simulink model "gimbal_test_2017_11_24"  (R2017a)
settings: Solver=ode14x  StartTime=0.0  StopTime=20  FixedStep=0.001  RelTol=1e-3  EnableMultiTasking=on
values from neighbouring files (symbols this model uses):
  m = MAG(:,3:5)    [acc_calibration_t1.m]
  s = tf('s')    [adaptive_control.m]    (also in constraints.m = 1e-19)
undefined symbols (not defined in the file or in its folder): sigbuilder_block, X, Y, Z
libraries: sm_lib x46, nesl_utility x35, simulink x7
(part 1 of 2)
settings Model: Creator=Chaohua Zhao  LastModifiedBy=Chaohua Zhao
settings DataIOCC: LimitDataPoints=on
settings OptimizationCC: LifeSpan=inf
settings DebuggingCC: AllowSymbolicDim=off  SFUnexpectedBacktrackingDiag=warning  SFNoUnconditionalDefaultTransitionDiag=warning  SFExecutionAtInitializationDiag=none
settings ModelReferenceCC: PropagateSignalLabelsOutOfModel=off
settings GRTTargetCC: TargetLangStandard=C89/C90 (ANSI)
settings ConfigComp: CovMetricSettings=dw  CovHtmlReporting=on  CovSaveCumulativeToWorkspaceVar=on  CovSaveSingleToWorkspaceVar=on  CovExternalEMLEnable=off
settings ConfigurationSet: Description=SimMechanics 2G

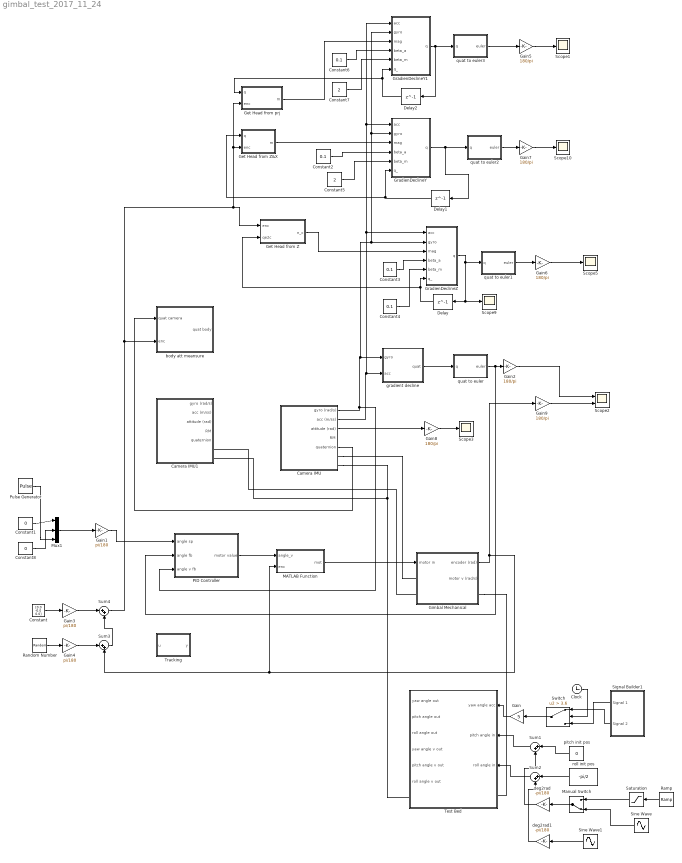
== system gimbal_test_2017_11_24 ==
  Camera IMU : Subsystem
  Camera IMU1 : Subsystem
  Clock : Clock
  Constant : Constant  Value=[0.0 -0.0 0.0]
  Constant1 : Constant  Value=0
  Constant{2..4,6} (4 alike) : Constant  Value=0.1
  Constant5 : Constant  Value=2
  Constant7 : Constant  Value=2
  Constant8 : Constant  Value=0
  Delay : Delay  DelayLength=1  InitialCondition=[1;0;0;0]
  Delay1 : Delay  DelayLength=1  InitialCondition=[1;0;0;0]
  Delay2 : Delay  DelayLength=1  InitialCondition=[1;0;0;0]
  Gain : Gain  Gain=5
  Gain1 : Gain  Gain=pi/180
  Gain{2,5..9} (6 alike) : Gain  Gain=180/pi
  Gain3 : Gain  Gain=pi/180
  Gain4 : Gain  Gain=pi/180
  Get Head from Z : MATLAB Function  TreatAsAtomicUnit=on
  Get Head from Z&X : MATLAB Function  TreatAsAtomicUnit=on
  "Get Head from prj " : MATLAB Function  TreatAsAtomicUnit=on
  Gimbal Mechanical : Subsystem
  GradienDeclineY : MATLAB Function  TreatAsAtomicUnit=on
  GradienDeclineY1 : MATLAB Function  TreatAsAtomicUnit=on
  GradienDeclineZ : MATLAB Function  TreatAsAtomicUnit=on
  MATLAB Function : MATLAB Function  TreatAsAtomicUnit=on
  Manual Switch : ManualSwitch  CurrentSetting=0
  Mux1 : Mux  Inputs=3
  PID Controller : Subsystem  TreatAsAtomicUnit=on
  Pulse Generator : DiscretePulseGenerator  PulseType=Time based  Amplitude=90  Period=3  PulseWidth=50
  Ramp : simulink/Sources/Ramp  slope=70  start=1  X0=0
  Random Number : RandomNumber  Variance=0.01  SampleTime=0.001
  Saturation : Saturate  UpperLimit=100  LowerLimit=-70
  Scope{1,3,5,9..10} (5 alike) : Scope
  Scope2 : Scope  NumInputPorts=2
  Signal Builder1 : Subsystem  Tag=STV Subsys  LoadFcn=sigbuilder_block('load');  StartFcn=sigbuilder_block('start');  StopFcn=sigbuilder_block('stop');  ClipboardFcn=sigbuilder_block('clipboard');  mask(Sigbuilder block){tuvar=[0:10]}
      mask help: Simulink:masks:SigbuilderBlock_MD
      mask init:
      | if ~strcmp(get_param(bdroot(gcbh),'SimulationStatus'),'stopped') tuvar = sigbuilder_block('maskInit'); end
      settings: CopyFcn=sigbuilder_block('copy');  DeleteFcn=sigbuilder_block('delete');  ModelCloseFcn=sigbuilder_block('modelClose');  PreSaveFcn=sigbuilder_block('preSave');  PauseFcn=sigbuilder_block('pause');  ContinueFcn=sigbuilder_block('continue');  NameChangeFcn=sigbuilder_block('namechange');  OpenFcn=sigbuilder_block('open',[6 74.25 1188 459 ]);  CloseFcn=sigbuilder_block('close');
      mask Display: plot(0, 0, 100, 100,[2, 2, 32, 32, 2], [68, 8, 8, 68, 68],[32, 2], [38, 38], [32, 19, 2],[53, 60, 44], [32, 17, 17, 2],[16, 16, 31, 31]);txt = getActiveGroup(gcbh);text(2, 100, txt,'verticalAlignment', 'top');
  Sine Wave : Sin  Amplitude=60  SampleTime=0
  Sine Wave1 : Sin  Amplitude=60  Frequency=1.7  SampleTime=0
  Sum{1..4} (4 alike) : Sum  Inputs=|++
  Switch : Switch  Criteria=u2 > Threshold  Threshold=3.6
  Test Bed : Subsystem
  Tracking : MATLAB Function  TreatAsAtomicUnit=on
  body att meansure : Subsystem
  deg2rad : Gain  Gain=-pi/180
  deg2rad1 : Gain  Gain=-pi/180
  gradient decline : Subsystem
  pitch init pos : Constant  Value=0
  quat to euler : MATLAB Function  TreatAsAtomicUnit=on
  quat to euler1 : MATLAB Function  TreatAsAtomicUnit=on
  quat to euler2 : MATLAB Function  TreatAsAtomicUnit=on
  quat to euler3 : MATLAB Function  TreatAsAtomicUnit=on
  roll init pos : Constant  Value=-pi/2
  wires:
  pitch init pos/1 -> Sum1/1
  roll init pos/1 -> Sum2/1
  Ramp/1 -> Saturation/1
  Saturation/1 -> Manual Switch/1
  Sine Wave/1 -> Manual Switch/2
  Manual Switch/1 -> deg2rad/1
  Clock/1 -> Switch/2
  Signal Builder1/2(Signal 2) -> Switch/1
  Signal Builder1/1(Signal 1) -> Switch/3
  Sum1/1 -> Test Bed/2(pitch angle in)
  Sum2/1 -> Test Bed/3(roll angle in)
  Sine Wave1/1 -> deg2rad1/1
  Gimbal Mechanical/1(encoder (rad)) -> Gain9/1, MATLAB Function/2(enc), Sum3/2
  Camera IMU/1(gyro (rad/s)) -> GradienDeclineY/2(gyro), GradienDeclineY1/2(gyro), GradienDeclineZ/2(gyro), gradient decline/1(gyro), PID Controller/3(angle v fb)
  Sum3/1 -> Sum4/2
  Constant/1 -> Gain3/1
  Gain3/1 -> Sum4/1
  Random Number/1 -> Gain4/1
  Gain4/1 -> Sum3/1
  Sum4/1 -> Get Head from Z/1(enc), "Get Head from prj "/2(enc), Get Head from Z&X/2(enc), body att meansure/2(enc)
  Camera IMU/2(acc (m/ss)) -> GradienDeclineY/1(acc), GradienDeclineY1/1(acc), GradienDeclineZ/1(acc), gradient decline/2(acc)
  gradient decline/1(quat) -> quat to euler/1(q)
  Camera IMU/5("quaternion ") -> body att meansure/1(quat camera)
  Gain1/1 -> PID Controller/1(angle sp)
  Gain2/1 -> Scope2/1
  GradienDeclineZ/1(q) -> quat to euler1/1(q), Delay/1, Scope9/1
  Delay/1 -> GradienDeclineZ/6(q_), Get Head from Z/2(qe2c)
  Constant3/1 -> GradienDeclineZ/4(beta_a)
  Switch/1 -> Gain/1
  Gain6/1 -> Scope5/1
  quat to euler1/1(euler) -> Gain6/1
  Get Head from Z/1(n_c) -> GradienDeclineZ/3(mag)
  Gain/1 -> Test Bed/1(yaw angle acc)
  Constant4/1 -> GradienDeclineZ/5(beta_m)
  Get Head from Z&X/1(m) -> GradienDeclineY/3(mag)
  Constant5/1 -> GradienDeclineY/5(beta_m)
  Constant2/1 -> GradienDeclineY/4(beta_a)
  Delay1/1 -> Get Head from Z&X/1(q), GradienDeclineY/6(q_)
  GradienDeclineY/1(q) -> quat to euler2/1(q), Delay1/1
  quat to euler2/1(euler) -> Gain7/1
  Gain7/1 -> Scope10/1
  quat to euler/1(euler) -> PID Controller/2(angle fb), Gain2/1
  "Get Head from prj "/1(m) -> GradienDeclineY1/3(mag)
  Constant6/1 -> GradienDeclineY1/4(beta_a)
  Constant7/1 -> GradienDeclineY1/5(beta_m)
  GradienDeclineY1/1(q) -> quat to euler3/1(q), Delay2/1
  Delay2/1 -> "Get Head from prj "/1(q), GradienDeclineY1/6(q_)
  Gain5/1 -> Scope1/1
  quat to euler3/1(euler) -> Gain5/1
  deg2rad/1 -> Sum1/2
  Gain8/1 -> Scope3/1
  Camera IMU/3(attitude (rad)) -> Gain8/1
  deg2rad1/1 -> Sum2/2
  Gain9/1 -> Scope2/2
  Constant1/1 -> Mux1/1
  Constant8/1 -> Mux1/2
  Pulse Generator/1 -> Mux1/3
  Mux1/1 -> Gain1/1
  PID Controller/1(motor value) -> MATLAB Function/1(angle_v)
  MATLAB Function/1(mot) -> Gimbal Mechanical/1(motor in)
  connections:
  Gimbal Mechanical/RConn1 -- Test Bed/LConn1
  Camera IMU/RConn1 -- Gimbal Mechanical/LConn1
  Camera IMU/RConn2 -- Camera IMU1/RConn2 -- Test Bed/RConn1
  Gimbal Mechanical/LConn2 -- Camera IMU1/RConn1

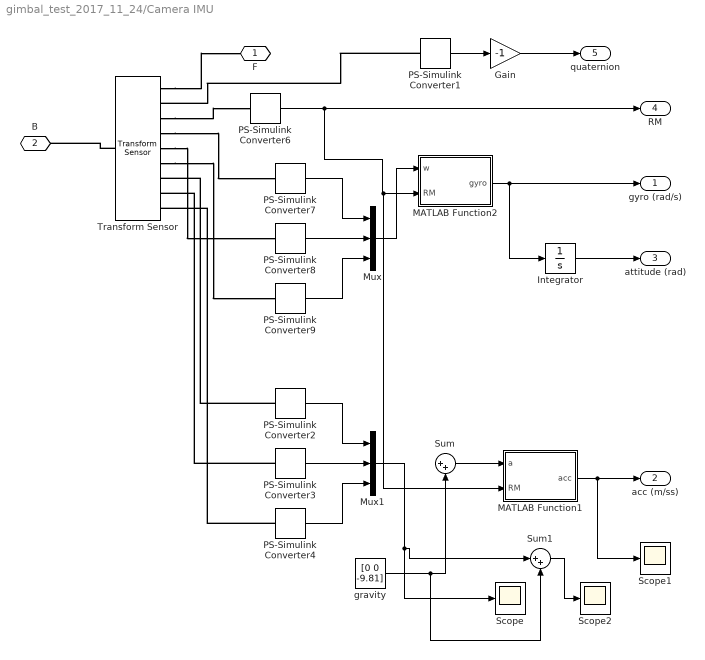
== system gimbal_test_2017_11_24/Camera IMU ==
  Gain : Gain  Gain=-1
  Integrator : Integrator
  MATLAB Function1 : MATLAB Function  TreatAsAtomicUnit=on
  MATLAB Function2 : MATLAB Function  TreatAsAtomicUnit=on
  Mux : Mux  Inputs=3
  Mux1 : Mux  Inputs=3
  PS-Simulink Converter{1..4,6..9} (8 alike) : nesl_utility/PS-Simulink Converter  PhysicalDomain=network_engine_domain  SubClassName=ps_output  LeftPortType=input  RightPortType=output  PseudoPeriodic=off  Frequencies=[]  Unit=1  AffineConversion=off
  Scope : Scope
  Scope1 : Scope
  Scope2 : Scope
  Sum : Sum  Inputs=|++
  Sum1 : Sum  Inputs=|++
  Transform Sensor : sm_lib/Frames and Transforms/Transform Sensor  MeasurementFrame=World  SenseAngle=off  SenseAxis=off  SenseAngle1=off  SenseAngle2=off  SenseAngle3=off  SenseQ=on  SenseR=on  SenseOmegaX=on  SenseOmegaY=on  SenseOmegaZ=on  SenseOmega1=off  SenseOmega2=off  SenseOmega3=off  SenseQDot=off  SenseRDot=off  SenseAlphaX=off  SenseAlphaY=off  SenseAlphaZ=off  SenseAlpha1=off  SenseAlpha2=off  SenseAlpha3=off  SenseQDDot=off  SenseRDDot=off  SenseX=off  SenseY=off  SenseZ=off  SenseRad=off  SenseAzim=off  SenseDist=off  SenseInc=off  SenseXDot=off  SenseYDot=off  SenseZDot=off  SenseRadDot=off  SenseAzimDot=off  SenseDistDot=off  SenseIncDot=off  SenseXDDot=on  SenseYDDot=on  SenseZDDot=on  SenseRadDDot=off  SenseAzimDDot=off  SenseDistDDot=off  SenseIncDDot=off
  "gravity " : Constant  Value=[0 0 -9.81]
  F : PMIOPort  Port=1  Side=Right
  B : PMIOPort  Port=2  Side=Right
  gyro (rad/s) : Outport
  acc (m/ss) : Outport  Port=2
  attitude (rad) : Outport  Port=3
  RM : Outport  Port=4
  "quaternion " : Outport  Port=5
  wires:
  PS-Simulink Converter6/1 -> RM/1, MATLAB Function1/2(RM), MATLAB Function2/2(RM)
  PS-Simulink Converter7/1 -> Mux/1
  PS-Simulink Converter9/1 -> Mux/3
  MATLAB Function2/1(gyro) -> gyro (rad/s)/1, Integrator/1
  PS-Simulink Converter8/1 -> Mux/2
  Integrator/1 -> attitude (rad)/1
  Mux/1 -> MATLAB Function2/1(w)
  PS-Simulink Converter1/1 -> Gain/1
  Gain/1 -> "quaternion "/1
  PS-Simulink Converter3/1 -> Mux1/2
  PS-Simulink Converter4/1 -> Mux1/3
  PS-Simulink Converter2/1 -> Mux1/1
  MATLAB Function1/1(acc) -> Scope1/1, acc (m/ss)/1
  "gravity "/1 -> Sum/2, Sum1/2
  Sum/1 -> MATLAB Function1/1(a)
  Sum1/1 -> Scope2/1
  Mux1/1 -> Sum1/1, Scope/1
  connections:
  Transform Sensor/LConn1 -- B/RConn1
  Transform Sensor/RConn1 -- F/RConn1
  Transform Sensor/RConn6 -- PS-Simulink Converter9/LConn1
  Transform Sensor/RConn5 -- PS-Simulink Converter8/LConn1
  Transform Sensor/RConn4 -- PS-Simulink Converter7/LConn1
  Transform Sensor/RConn3 -- PS-Simulink Converter6/LConn1
  PS-Simulink Converter1/LConn1 -- Transform Sensor/RConn2
  PS-Simulink Converter3/LConn1 -- Transform Sensor/RConn8
  PS-Simulink Converter4/LConn1 -- Transform Sensor/RConn9
  PS-Simulink Converter2/LConn1 -- Transform Sensor/RConn7

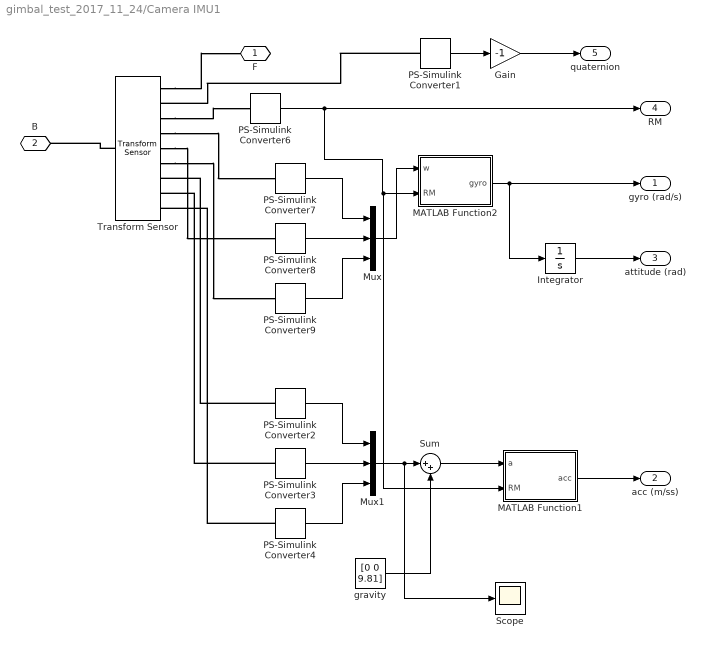
== system gimbal_test_2017_11_24/Camera IMU1 ==
  Gain : Gain  Gain=-1
  Integrator : Integrator
  MATLAB Function1 : MATLAB Function  TreatAsAtomicUnit=on
  MATLAB Function2 : MATLAB Function  TreatAsAtomicUnit=on
  Mux : Mux  Inputs=3
  Mux1 : Mux  Inputs=3
  PS-Simulink Converter{1..4,6..9} (8 alike) : nesl_utility/PS-Simulink Converter  PhysicalDomain=network_engine_domain  SubClassName=ps_output  LeftPortType=input  RightPortType=output  PseudoPeriodic=off  Frequencies=[]  Unit=1  AffineConversion=off
  Scope : Scope
  Sum : Sum  Inputs=|++
  Transform Sensor : sm_lib/Frames and Transforms/Transform Sensor  MeasurementFrame=World  SenseAngle=off  SenseAxis=off  SenseAngle1=off  SenseAngle2=off  SenseAngle3=off  SenseQ=on  SenseR=on  SenseOmegaX=on  SenseOmegaY=on  SenseOmegaZ=on  SenseOmega1=off  SenseOmega2=off  SenseOmega3=off  SenseQDot=off  SenseRDot=off  SenseAlphaX=off  SenseAlphaY=off  SenseAlphaZ=off  SenseAlpha1=off  SenseAlpha2=off  SenseAlpha3=off  SenseQDDot=off  SenseRDDot=off  SenseX=off  SenseY=off  SenseZ=off  SenseRad=off  SenseAzim=off  SenseDist=off  SenseInc=off  SenseXDot=off  SenseYDot=off  SenseZDot=off  SenseRadDot=off  SenseAzimDot=off  SenseDistDot=off  SenseIncDot=off  SenseXDDot=on  SenseYDDot=on  SenseZDDot=on  SenseRadDDot=off  SenseAzimDDot=off  SenseDistDDot=off  SenseIncDDot=off
  "gravity " : Constant  Value=[0 0 9.81]
  F : PMIOPort  Port=1  Side=Right
  B : PMIOPort  Port=2  Side=Right
  gyro (rad/s) : Outport
  acc (m/ss) : Outport  Port=2
  attitude (rad) : Outport  Port=3
  RM : Outport  Port=4
  "quaternion " : Outport  Port=5
  wires:
  Sum/1 -> MATLAB Function1/1(a)
  "gravity "/1 -> Sum/2
  Mux1/1 -> Sum/1, Scope/1
  MATLAB Function1/1(acc) -> acc (m/ss)/1
  PS-Simulink Converter2/1 -> Mux1/1
  PS-Simulink Converter4/1 -> Mux1/3
  PS-Simulink Converter3/1 -> Mux1/2
  Gain/1 -> "quaternion "/1
  PS-Simulink Converter1/1 -> Gain/1
  Mux/1 -> MATLAB Function2/1(w)
  Integrator/1 -> attitude (rad)/1
  PS-Simulink Converter8/1 -> Mux/2
  MATLAB Function2/1(gyro) -> Integrator/1, gyro (rad/s)/1
  PS-Simulink Converter9/1 -> Mux/3
  PS-Simulink Converter7/1 -> Mux/1
  PS-Simulink Converter6/1 -> MATLAB Function2/2(RM), MATLAB Function1/2(RM), RM/1
  connections:
  PS-Simulink Converter2/LConn1 -- Transform Sensor/RConn7
  PS-Simulink Converter4/LConn1 -- Transform Sensor/RConn9
  PS-Simulink Converter3/LConn1 -- Transform Sensor/RConn8
  PS-Simulink Converter1/LConn1 -- Transform Sensor/RConn2
  Transform Sensor/RConn3 -- PS-Simulink Converter6/LConn1
  Transform Sensor/RConn4 -- PS-Simulink Converter7/LConn1
  Transform Sensor/RConn5 -- PS-Simulink Converter8/LConn1
  Transform Sensor/RConn6 -- PS-Simulink Converter9/LConn1
  Transform Sensor/RConn1 -- F/RConn1
  Transform Sensor/LConn1 -- B/RConn1

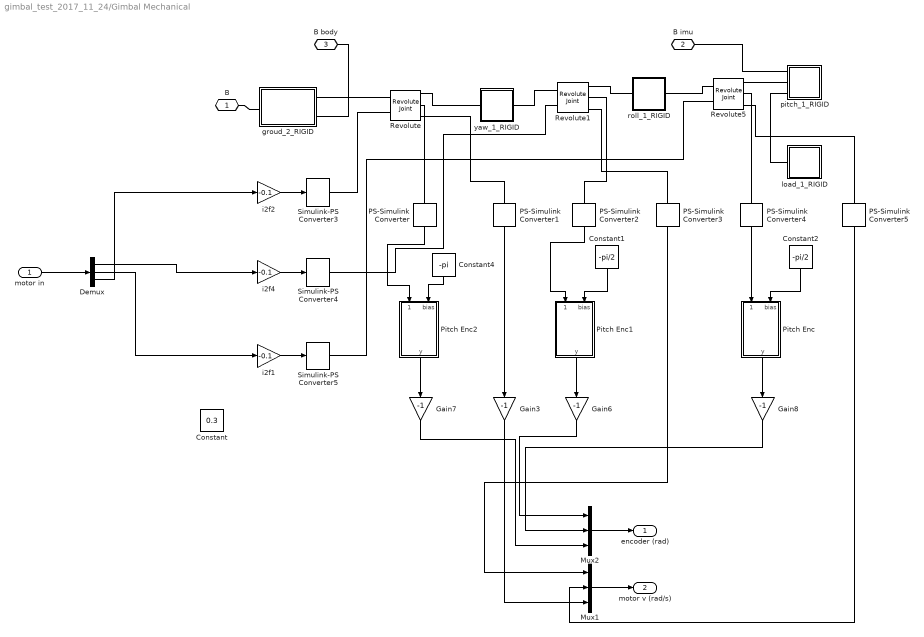
== system gimbal_test_2017_11_24/Gimbal Mechanical ==
  motor in : Inport
  Constant : Constant  Value=0.3
  Constant1 : Constant  Value=-pi/2
  Constant2 : Constant  Value=-pi/2
  Constant4 : Constant  Value=-pi
  Demux : Demux  Outputs=3
  Gain{3,6..8} (4 alike) : Gain  Gain=-1
  Mux1 : Mux  Inputs=3
  Mux2 : Mux  Inputs=3
  PS-Simulink Converter{,1..5} (6 alike) : nesl_utility/PS-Simulink Converter  PhysicalDomain=network_engine_domain  SubClassName=ps_output  LeftPortType=input  RightPortType=output  PseudoPeriodic=off  Frequencies=[]  Unit=1  AffineConversion=off
  Pitch Enc : MATLAB Function  TreatAsAtomicUnit=on
  Pitch Enc1 : MATLAB Function  TreatAsAtomicUnit=on
  Pitch Enc2 : MATLAB Function  TreatAsAtomicUnit=on
  Revolute : sm_lib/Joints/Revolute Joint  SenseConstraintForce=off  SenseConstraintForceX=off  SenseConstraintForceY=off  SenseConstraintForceZ=off  SenseConstraintTorque=off  SenseConstraintTorqueX=off  SenseConstraintTorqueY=off  SenseConstraintTorqueZ=off  SenseTotalForce=off  SenseTotalForceX=off  SenseTotalForceY=off  SenseTotalForceZ=off  SenseTotalTorque=off  SenseTotalTorqueX=off  SenseTotalTorqueY=off  SenseTotalTorqueZ=off  CompositeWrenchDir=FollowerOnBase  CompositeWrenchFrame=BaseFrame  EquilibriumPosition=0  EquilibriumPositionUnits=rad  SpringStiffness=0  SpringStiffnessUnits=m*N/rad  DampingCoefficient=0  DampingCoefficientUnits=m*s*N/rad  TorqueActuationMode=InputTorque  MotionActuationMode=ComputedMotion  SensePosition=on  SenseVelocity=on  SenseAcceleration=off  SenseTorqueForce=off  PositionTargetSpecify=on  PositionTargetPriority=Low  PositionTargetValue=180  PositionTargetValueUnits=deg  VelocityTargetSpecify=off  VelocityTargetPriority=High  VelocityTargetValue=0  VelocityTargetValueUnits=deg/s
  Revolute1 : sm_lib/Joints/Revolute Joint  SenseConstraintForce=off  SenseConstraintForceX=off  SenseConstraintForceY=off  SenseConstraintForceZ=off  SenseConstraintTorque=off  SenseConstraintTorqueX=off  SenseConstraintTorqueY=off  SenseConstraintTorqueZ=off  SenseTotalForce=off  SenseTotalForceX=off  SenseTotalForceY=off  SenseTotalForceZ=off  SenseTotalTorque=off  SenseTotalTorqueX=off  SenseTotalTorqueY=off  SenseTotalTorqueZ=off  CompositeWrenchDir=FollowerOnBase  CompositeWrenchFrame=BaseFrame  EquilibriumPosition=0  EquilibriumPositionUnits=rad  SpringStiffness=0  SpringStiffnessUnits=m*N/rad  DampingCoefficient=0  DampingCoefficientUnits=m*s*N/rad  TorqueActuationMode=InputTorque  MotionActuationMode=ComputedMotion  SensePosition=on  SenseVelocity=on  SenseAcceleration=off  SenseTorqueForce=off  PositionTargetSpecify=on  PositionTargetPriority=Low  PositionTargetValue=90  PositionTargetValueUnits=deg  VelocityTargetSpecify=off  VelocityTargetPriority=High  VelocityTargetValue=0  VelocityTargetValueUnits=deg/s
  Revolute5 : sm_lib/Joints/Revolute Joint  SenseConstraintForce=off  SenseConstraintForceX=off  SenseConstraintForceY=off  SenseConstraintForceZ=off  SenseConstraintTorque=off  SenseConstraintTorqueX=off  SenseConstraintTorqueY=off  SenseConstraintTorqueZ=off  SenseTotalForce=off  SenseTotalForceX=off  SenseTotalForceY=off  SenseTotalForceZ=off  SenseTotalTorque=off  SenseTotalTorqueX=off  SenseTotalTorqueY=off  SenseTotalTorqueZ=off  CompositeWrenchDir=FollowerOnBase  CompositeWrenchFrame=BaseFrame  EquilibriumPosition=0  EquilibriumPositionUnits=rad  SpringStiffness=0  SpringStiffnessUnits=m*N/rad  DampingCoefficient=0  DampingCoefficientUnits=m*s*N/rad  TorqueActuationMode=InputTorque  MotionActuationMode=ComputedMotion  SensePosition=on  SenseVelocity=on  SenseAcceleration=off  SenseTorqueForce=off  PositionTargetSpecify=on  PositionTargetPriority=Low  PositionTargetValue=90  PositionTargetValueUnits=deg  VelocityTargetSpecify=off  VelocityTargetPriority=High  VelocityTargetValue=0  VelocityTargetValueUnits=deg/s
  Simulink-PS Converter3 : nesl_utility/Simulink-PS Converter  PhysicalDomain=network_engine_domain  SubClassName=ps_input  LeftPortType=input  RightPortType=output  PseudoPeriodic=off  Frequencies=[]  NoiseDistribution=none  NoiseParameters=[]  Unit=1  AffineConversion=off  FilteringAndDerivatives=zero  SimscapeFilterOrder=1  InputFilterTimeConstant=0.001  UdotUserProvided=1
  Simulink-PS Converter4 : nesl_utility/Simulink-PS Converter  PhysicalDomain=network_engine_domain  SubClassName=ps_input  LeftPortType=input  RightPortType=output  PseudoPeriodic=off  Frequencies=[]  NoiseDistribution=none  NoiseParameters=[]  Unit=1  AffineConversion=off  FilteringAndDerivatives=zero  SimscapeFilterOrder=1  InputFilterTimeConstant=0.001  UdotUserProvided=1
  Simulink-PS Converter5 : nesl_utility/Simulink-PS Converter  PhysicalDomain=network_engine_domain  SubClassName=ps_input  LeftPortType=input  RightPortType=output  PseudoPeriodic=off  Frequencies=[]  NoiseDistribution=none  NoiseParameters=[]  Unit=1  AffineConversion=off  FilteringAndDerivatives=zero  SimscapeFilterOrder=1  InputFilterTimeConstant=0.001  UdotUserProvided=1
  groud_2_RIGID : Subsystem
  i2f1 : Gain  Gain=-0.1
  i2f2 : Gain  Gain=-0.1
  i2f4 : Gain  Gain=-0.1
  load_1_RIGID : Subsystem
  pitch_1_RIGID : Subsystem
  roll_1_RIGID : Subsystem
  yaw_1_RIGID : Subsystem
  B : PMIOPort  Port=1  Side=Right
  B imu : PMIOPort  Port=2  Side=Left
  B body : PMIOPort  Port=3  Side=Left
  encoder (rad) : Outport
  motor v (rad/s) : Outport  Port=2
  wires:
  PS-Simulink Converter5/1 -> Mux1/2
  PS-Simulink Converter2/1 -> Pitch Enc1/1(angle)
  Constant1/1 -> Pitch Enc1/2(bias)
  Constant4/1 -> Pitch Enc2/2(bias)
  PS-Simulink Converter1/1 -> Gain3/1
  Constant2/1 -> Pitch Enc/2(bias)
  PS-Simulink Converter/1 -> Pitch Enc2/1(angle)
  PS-Simulink Converter4/1 -> Pitch Enc/1(angle)
  Pitch Enc1/1(y) -> Gain6/1
  Pitch Enc/1(y) -> Gain8/1
  PS-Simulink Converter3/1 -> Mux1/1
  Pitch Enc2/1(y) -> Gain7/1
  Gain7/1 -> Mux2/3
  Gain8/1 -> Mux2/2
  i2f4/1 -> Simulink-PS Converter4/1
  i2f1/1 -> Simulink-PS Converter5/1
  i2f2/1 -> Simulink-PS Converter3/1
  Gain6/1 -> Mux2/1
  ? -> ?
  Mux2/1 -> encoder (rad)/1
  Mux1/1 -> motor v (rad/s)/1
  Gain3/1 -> Mux1/3
  motor in/1 -> Demux/1
  Demux/1 -> i2f4/1
  Demux/2 -> i2f1/1
  Demux/3 -> i2f2/1
  connections:
  Revolute5/RConn1 -- pitch_1_RIGID/LConn2
  Revolute1/LConn1 -- yaw_1_RIGID/RConn1
  Revolute1/RConn1 -- roll_1_RIGID/LConn1
  Revolute/LConn1 -- groud_2_RIGID/RConn1
  groud_2_RIGID/LConn1 -- B/RConn1
  Revolute/RConn1 -- yaw_1_RIGID/LConn1
  load_1_RIGID/LConn1 -- pitch_1_RIGID/LConn3
  Revolute5/LConn1 -- roll_1_RIGID/RConn1
  Simulink-PS Converter5/RConn1 -- Revolute5/LConn2
  PS-Simulink Converter4/LConn1 -- Revolute5/RConn2
  PS-Simulink Converter5/LConn1 -- Revolute5/RConn3
  PS-Simulink Converter/LConn1 -- Revolute/RConn2
  PS-Simulink Converter3/LConn1 -- Revolute1/RConn3
  PS-Simulink Converter2/LConn1 -- Revolute1/RConn2
  PS-Simulink Converter1/LConn1 -- Revolute/RConn3
  Simulink-PS Converter3/RConn1 -- Revolute/LConn2
  Simulink-PS Converter4/RConn1 -- Revolute1/LConn2
  B imu/RConn1 -- pitch_1_RIGID/LConn1
  groud_2_RIGID/RConn2 -- B body/RConn1

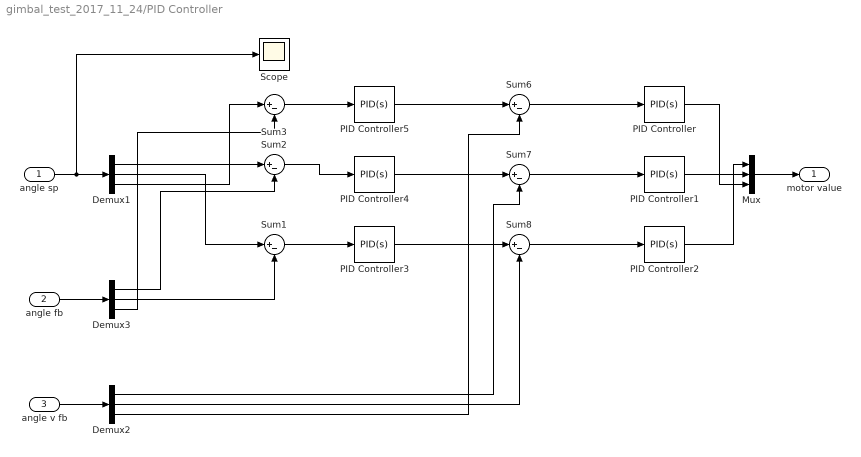
== system gimbal_test_2017_11_24/PID Controller ==
  angle sp : Inport
  angle fb : Inport  Port=2
  angle v fb : Inport  Port=3
  Demux1 : Demux  Outputs=3
  Demux2 : Demux  Outputs=3
  Demux3 : Demux  Outputs=3
  Mux : Mux  Inputs=3
  PID Controller : simulink/Continuous/PID Controller  Controller=PID  TimeDomain=Continuous-time  SampleTime=-1  IntegratorMethod=Forward Euler  FilterMethod=Forward Euler  Form=Parallel  UseFilter=on  ControllerParametersSource=internal  P=50  I=2  D=0.5  N=1  InitialConditionSource=internal  InitialConditionForIntegrator=0  InitialConditionForFilter=0  ExternalReset=none  LimitOutput=on  UpperSaturationLimit=10  LowerSaturationLimit=-10  LinearizeAsGain=on  AntiWindupMode=none  Kb=1  TrackingMode=off  Kt=1  PParamMin=[]  PParamMax=[]  IParamMin=[]  IParamMax=[]  DParamMin=[]  DParamMax=[]  NParamMin=[]  NParamMax=[]  KbParamMin=[]  KbParamMax=[]  KtParamMin=[]  KtParamMax=[]  POutMin=[]  POutMax=[]  IOutMin=[]  IOutMax=[]  DOutMin=[]  DOutMax=[]  NOutMin=[]  NOutMax=[]  KbOutMin=[]  KbOutMax=[]  KtOutMin=[]  KtOutMax=[]  IntegratorOutMin=[]  IntegratorOutMax=[]  FilterOutMin=[]  FilterOutMax=[]  SumOutMin=[]  SumOutMax=[]  SumI1OutMin=[]  SumI1OutMax=[]  SumI2OutMin=[]  SumI2OutMax=[]  SumI3OutMin=[]  SumI3OutMax=[]  SumDOutMin=[]  SumDOutMax=[]  SaturationOutMin=[]  SaturationOutMax=[]  IntegratorContinuousStateAttributes=''  IntegratorStateMustResolveToSignalObject=off  IntegratorRTWStateStorageClass=Auto  FilterContinuousStateAttributes=''  FilterStateMustResolveToSignalObject=off  FilterRTWStateStorageClass=Auto  DifferentiatorICPrevScaledInput=0  DifferentiatorOutMin=[]  DifferentiatorOutMax=[]  InitialConditionSetting=State (most efficient)
  PID Controller1 : simulink/Continuous/PID Controller  Controller=PID  TimeDomain=Continuous-time  SampleTime=-1  IntegratorMethod=Forward Euler  FilterMethod=Forward Euler  Form=Parallel  UseFilter=on  ControllerParametersSource=internal  P=50  I=2  D=0.5  N=20  InitialConditionSource=internal  InitialConditionForIntegrator=0  InitialConditionForFilter=0  ExternalReset=none  LimitOutput=on  UpperSaturationLimit=10  LowerSaturationLimit=-10  LinearizeAsGain=on  AntiWindupMode=none  Kb=1  TrackingMode=off  Kt=1  PParamMin=[]  PParamMax=[]  IParamMin=[]  IParamMax=[]  DParamMin=[]  DParamMax=[]  NParamMin=[]  NParamMax=[]  KbParamMin=[]  KbParamMax=[]  KtParamMin=[]  KtParamMax=[]  POutMin=[]  POutMax=[]  IOutMin=[]  IOutMax=[]  DOutMin=[]  DOutMax=[]  NOutMin=[]  NOutMax=[]  KbOutMin=[]  KbOutMax=[]  KtOutMin=[]  KtOutMax=[]  IntegratorOutMin=[]  IntegratorOutMax=[]  FilterOutMin=[]  FilterOutMax=[]  SumOutMin=[]  SumOutMax=[]  SumI1OutMin=[]  SumI1OutMax=[]  SumI2OutMin=[]  SumI2OutMax=[]  SumI3OutMin=[]  SumI3OutMax=[]  SumDOutMin=[]  SumDOutMax=[]  SaturationOutMin=[]  SaturationOutMax=[]  IntegratorContinuousStateAttributes=''  IntegratorStateMustResolveToSignalObject=off  IntegratorRTWStateStorageClass=Auto  FilterContinuousStateAttributes=''  FilterStateMustResolveToSignalObject=off  FilterRTWStateStorageClass=Auto  DifferentiatorICPrevScaledInput=0  DifferentiatorOutMin=[]  DifferentiatorOutMax=[]  InitialConditionSetting=State (most efficient)
  PID Controller2 : simulink/Continuous/PID Controller  Controller=PID  TimeDomain=Continuous-time  SampleTime=-1  IntegratorMethod=Forward Euler  FilterMethod=Forward Euler  Form=Parallel  UseFilter=on  ControllerParametersSource=internal  P=50  I=0.4  D=0.5  N=20  InitialConditionSource=internal  InitialConditionForIntegrator=0  InitialConditionForFilter=0  ExternalReset=none  LimitOutput=on  UpperSaturationLimit=10  LowerSaturationLimit=-10  LinearizeAsGain=on  AntiWindupMode=none  Kb=1  TrackingMode=off  Kt=1  PParamMin=[]  PParamMax=[]  IParamMin=[]  IParamMax=[]  DParamMin=[]  DParamMax=[]  NParamMin=[]  NParamMax=[]  KbParamMin=[]  KbParamMax=[]  KtParamMin=[]  KtParamMax=[]  POutMin=[]  POutMax=[]  IOutMin=[]  IOutMax=[]  DOutMin=[]  DOutMax=[]  NOutMin=[]  NOutMax=[]  KbOutMin=[]  KbOutMax=[]  KtOutMin=[]  KtOutMax=[]  IntegratorOutMin=[]  IntegratorOutMax=[]  FilterOutMin=[]  FilterOutMax=[]  SumOutMin=[]  SumOutMax=[]  SumI1OutMin=[]  SumI1OutMax=[]  SumI2OutMin=[]  SumI2OutMax=[]  SumI3OutMin=[]  SumI3OutMax=[]  SumDOutMin=[]  SumDOutMax=[]  SaturationOutMin=[]  SaturationOutMax=[]  IntegratorContinuousStateAttributes=''  IntegratorStateMustResolveToSignalObject=off  IntegratorRTWStateStorageClass=Auto  FilterContinuousStateAttributes=''  FilterStateMustResolveToSignalObject=off  FilterRTWStateStorageClass=Auto  DifferentiatorICPrevScaledInput=0  DifferentiatorOutMin=[]  DifferentiatorOutMax=[]  InitialConditionSetting=State (most efficient)
  PID Controller3 : simulink/Continuous/PID Controller  Controller=PID  TimeDomain=Continuous-time  SampleTime=-1  IntegratorMethod=Forward Euler  FilterMethod=Forward Euler  Form=Parallel  UseFilter=on  ControllerParametersSource=internal  P=10  I=0  D=0  N=20  InitialConditionSource=internal  InitialConditionForIntegrator=0  InitialConditionForFilter=0  ExternalReset=none  LimitOutput=on  UpperSaturationLimit=6  LowerSaturationLimit=-6  LinearizeAsGain=on  AntiWindupMode=none  Kb=1  TrackingMode=off  Kt=1  PParamMin=[]  PParamMax=[]  IParamMin=[]  IParamMax=[]  DParamMin=[]  DParamMax=[]  NParamMin=[]  NParamMax=[]  KbParamMin=[]  KbParamMax=[]  KtParamMin=[]  KtParamMax=[]  POutMin=[]  POutMax=[]  IOutMin=[]  IOutMax=[]  DOutMin=[]  DOutMax=[]  NOutMin=[]  NOutMax=[]  KbOutMin=[]  KbOutMax=[]  KtOutMin=[]  KtOutMax=[]  IntegratorOutMin=[]  IntegratorOutMax=[]  FilterOutMin=[]  FilterOutMax=[]  SumOutMin=[]  SumOutMax=[]  SumI1OutMin=[]  SumI1OutMax=[]  SumI2OutMin=[]  SumI2OutMax=[]  SumI3OutMin=[]  SumI3OutMax=[]  SumDOutMin=[]  SumDOutMax=[]  SaturationOutMin=[]  SaturationOutMax=[]  IntegratorContinuousStateAttributes=''  IntegratorStateMustResolveToSignalObject=off  IntegratorRTWStateStorageClass=Auto  FilterContinuousStateAttributes=''  FilterStateMustResolveToSignalObject=off  FilterRTWStateStorageClass=Auto  DifferentiatorICPrevScaledInput=0  DifferentiatorOutMin=[]  DifferentiatorOutMax=[]  InitialConditionSetting=State (most efficient)
  PID Controller4 : simulink/Continuous/PID Controller  Controller=PID  TimeDomain=Continuous-time  SampleTime=-1  IntegratorMethod=Forward Euler  FilterMethod=Forward Euler  Form=Parallel  UseFilter=on  ControllerParametersSource=internal  P=10  I=0  D=0  N=20  InitialConditionSource=internal  InitialConditionForIntegrator=0  InitialConditionForFilter=0  ExternalReset=none  LimitOutput=on  UpperSaturationLimit=6  LowerSaturationLimit=-6  LinearizeAsGain=on  AntiWindupMode=none  Kb=1  TrackingMode=off  Kt=1  PParamMin=[]  PParamMax=[]  IParamMin=[]  IParamMax=[]  DParamMin=[]  DParamMax=[]  NParamMin=[]  NParamMax=[]  KbParamMin=[]  KbParamMax=[]  KtParamMin=[]  KtParamMax=[]  POutMin=[]  POutMax=[]  IOutMin=[]  IOutMax=[]  DOutMin=[]  DOutMax=[]  NOutMin=[]  NOutMax=[]  KbOutMin=[]  KbOutMax=[]  KtOutMin=[]  KtOutMax=[]  IntegratorOutMin=[]  IntegratorOutMax=[]  FilterOutMin=[]  FilterOutMax=[]  SumOutMin=[]  SumOutMax=[]  SumI1OutMin=[]  SumI1OutMax=[]  SumI2OutMin=[]  SumI2OutMax=[]  SumI3OutMin=[]  SumI3OutMax=[]  SumDOutMin=[]  SumDOutMax=[]  SaturationOutMin=[]  SaturationOutMax=[]  IntegratorContinuousStateAttributes=''  IntegratorStateMustResolveToSignalObject=off  IntegratorRTWStateStorageClass=Auto  FilterContinuousStateAttributes=''  FilterStateMustResolveToSignalObject=off  FilterRTWStateStorageClass=Auto  DifferentiatorICPrevScaledInput=0  DifferentiatorOutMin=[]  DifferentiatorOutMax=[]  InitialConditionSetting=State (most efficient)
  PID Controller5 : simulink/Continuous/PID Controller  Controller=PID  TimeDomain=Continuous-time  SampleTime=-1  IntegratorMethod=Forward Euler  FilterMethod=Forward Euler  Form=Parallel  UseFilter=on  ControllerParametersSource=internal  P=10  I=0  D=0  N=1  InitialConditionSource=internal  InitialConditionForIntegrator=0  InitialConditionForFilter=0  ExternalReset=none  LimitOutput=on  UpperSaturationLimit=6  LowerSaturationLimit=-6  LinearizeAsGain=on  AntiWindupMode=none  Kb=1  TrackingMode=off  Kt=1  PParamMin=[]  PParamMax=[]  IParamMin=[]  IParamMax=[]  DParamMin=[]  DParamMax=[]  NParamMin=[]  NParamMax=[]  KbParamMin=[]  KbParamMax=[]  KtParamMin=[]  KtParamMax=[]  POutMin=[]  POutMax=[]  IOutMin=[]  IOutMax=[]  DOutMin=[]  DOutMax=[]  NOutMin=[]  NOutMax=[]  KbOutMin=[]  KbOutMax=[]  KtOutMin=[]  KtOutMax=[]  IntegratorOutMin=[]  IntegratorOutMax=[]  FilterOutMin=[]  FilterOutMax=[]  SumOutMin=[]  SumOutMax=[]  SumI1OutMin=[]  SumI1OutMax=[]  SumI2OutMin=[]  SumI2OutMax=[]  SumI3OutMin=[]  SumI3OutMax=[]  SumDOutMin=[]  SumDOutMax=[]  SaturationOutMin=[]  SaturationOutMax=[]  IntegratorContinuousStateAttributes=''  IntegratorStateMustResolveToSignalObject=off  IntegratorRTWStateStorageClass=Auto  FilterContinuousStateAttributes=''  FilterStateMustResolveToSignalObject=off  FilterRTWStateStorageClass=Auto  DifferentiatorICPrevScaledInput=0  DifferentiatorOutMin=[]  DifferentiatorOutMax=[]  InitialConditionSetting=State (most efficient)
  Scope : Scope
  Sum{1..3,6..8} (6 alike) : Sum  Inputs=|+-
  motor value : Outport
  wires:
  Demux2/2 -> Sum8/2
  Sum7/1 -> PID Controller1/1
  Demux2/3 -> Sum6/2
  Sum8/1 -> PID Controller2/1
  Demux2/1 -> Sum7/2
  Sum6/1 -> PID Controller/1
  PID Controller2/1 -> Mux/2
  PID Controller/1 -> Mux/3
  angle v fb/1 -> Demux2/1
  Mux/1 -> motor value/1
  PID Controller1/1 -> Mux/1
  angle sp/1 -> Scope/1, Demux1/1
  PID Controller5/1 -> Sum6/1
  PID Controller4/1 -> Sum7/1
  PID Controller3/1 -> Sum8/1
  Demux1/3 -> Sum3/1
  Sum3/1 -> PID Controller5/1
  Demux1/1 -> Sum2/1
  Sum2/1 -> PID Controller4/1
  Demux1/2 -> Sum1/1
  Sum1/1 -> PID Controller3/1
  Demux3/1 -> Sum2/2
  Demux3/2 -> Sum1/2
  Demux3/3 -> Sum3/2
  angle fb/1 -> Demux3/1

== system gimbal_test_2017_11_24/Signal Builder1 ==
  Demux : Demux  Tag=STV Demux  Outputs=2
  FromWs : FromWorkspace  Tag=STV FromWs  VariableName=tuvar  SampleTime=0
      SigBuilderData=|
      | common.afterFinalStr = 'Extrapolate'
      | common.sampleTime = 0
      | dataSet.timeRange = [0 10]
      | dataSet.name = 'Group 1'
      | sbobj.Groups.Name = 'Group 1'
      | sbobj.Groups.Signals(1).Name = 'Signal 1'
      | sbobj.Groups.Signals(1).XData = [0 2.9 3.1 3.2 3.4 10]
      | sbobj.Groups.Signals(1).YData = [0 0 1 1 -0.005 0]
      | sbobj.Groups.Signals(2).Name = 'Signal 2'
      | sbobj.Groups.Signals(2).XData = [0 3.9 4.1 4.2 4.4 10]
      | sbobj.Groups.Signals(2).YData = [0 0 -1 -1 0 0]
  Signal 1 : Outport  Tag=STV Outport
  Signal 2 : Outport  Tag=STV Outport  Port=2
  wires:
  Demux/1 -> Signal 1/1
  FromWs/1 -> Demux/1
  Demux/2 -> Signal 2/1

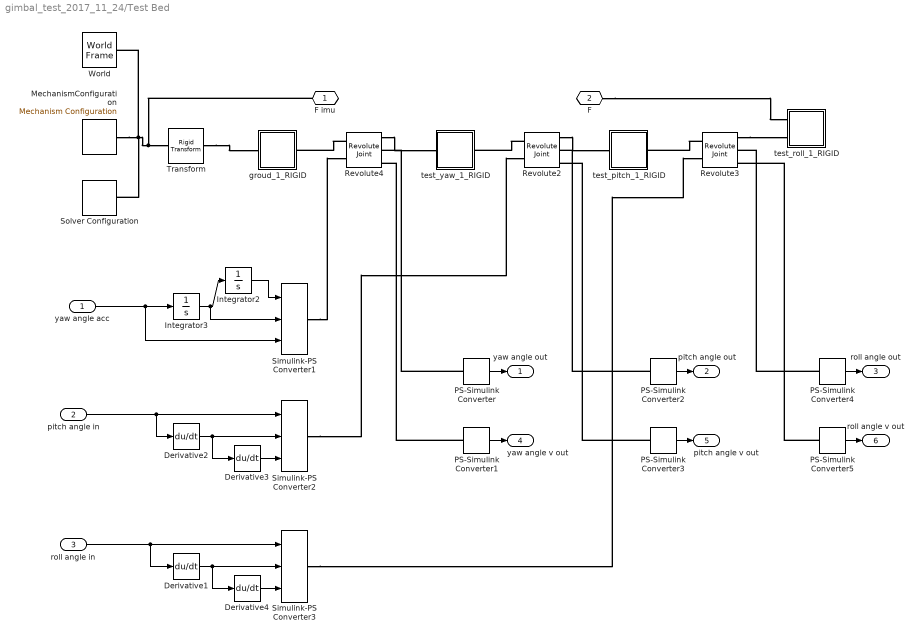
== system gimbal_test_2017_11_24/Test Bed ==
  yaw angle acc : Inport
  pitch angle in : Inport  Port=2
  roll angle in : Inport  Port=3
  Derivative{1..4} (4 alike) : Derivative
  Integrator2 : Integrator
  Integrator3 : Integrator
  MechanismConfiguration : sm_lib/Utilities/Mechanism Configuration  UniformGravity=Constant  GravityVector=[0 0 -9.81]  GravityUnits=m/s^2  LinearizationDelta=0.001
  PS-Simulink Converter{,1..5} (6 alike) : nesl_utility/PS-Simulink Converter  PhysicalDomain=network_engine_domain  SubClassName=ps_output  LeftPortType=input  RightPortType=output  PseudoPeriodic=off  Frequencies=[]  Unit=1  AffineConversion=off
  Revolute2 : sm_lib/Joints/Revolute Joint  SenseConstraintForce=off  SenseConstraintForceX=off  SenseConstraintForceY=off  SenseConstraintForceZ=off  SenseConstraintTorque=off  SenseConstraintTorqueX=off  SenseConstraintTorqueY=off  SenseConstraintTorqueZ=off  SenseTotalForce=off  SenseTotalForceX=off  SenseTotalForceY=off  SenseTotalForceZ=off  SenseTotalTorque=off  SenseTotalTorqueX=off  SenseTotalTorqueY=off  SenseTotalTorqueZ=off  CompositeWrenchDir=FollowerOnBase  CompositeWrenchFrame=BaseFrame  EquilibriumPosition=0  EquilibriumPositionUnits=rad  SpringStiffness=0  SpringStiffnessUnits=m*N/rad  DampingCoefficient=0  DampingCoefficientUnits=m*s*N/rad  TorqueActuationMode=ComputedTorque  MotionActuationMode=InputMotion  SensePosition=on  SenseVelocity=on  SenseAcceleration=off  SenseTorqueForce=off  PositionTargetSpecify=off  PositionTargetPriority=High  PositionTargetValue=0  PositionTargetValueUnits=deg  VelocityTargetSpecify=off  VelocityTargetPriority=High  VelocityTargetValue=0  VelocityTargetValueUnits=deg/s
  Revolute3 : sm_lib/Joints/Revolute Joint  SenseConstraintForce=off  SenseConstraintForceX=off  SenseConstraintForceY=off  SenseConstraintForceZ=off  SenseConstraintTorque=off  SenseConstraintTorqueX=off  SenseConstraintTorqueY=off  SenseConstraintTorqueZ=off  SenseTotalForce=off  SenseTotalForceX=off  SenseTotalForceY=off  SenseTotalForceZ=off  SenseTotalTorque=off  SenseTotalTorqueX=off  SenseTotalTorqueY=off  SenseTotalTorqueZ=off  CompositeWrenchDir=FollowerOnBase  CompositeWrenchFrame=BaseFrame  EquilibriumPosition=0  EquilibriumPositionUnits=rad  SpringStiffness=0  SpringStiffnessUnits=m*N/rad  DampingCoefficient=0  DampingCoefficientUnits=m*s*N/rad  TorqueActuationMode=ComputedTorque  MotionActuationMode=InputMotion  SensePosition=on  SenseVelocity=on  SenseAcceleration=off  SenseTorqueForce=off  PositionTargetSpecify=on  PositionTargetPriority=Low  PositionTargetValue=70.269058625743583  PositionTargetValueUnits=deg  VelocityTargetSpecify=off  VelocityTargetPriority=High  VelocityTargetValue=0  VelocityTargetValueUnits=deg/s
  Revolute4 : sm_lib/Joints/Revolute Joint  SenseConstraintForce=off  SenseConstraintForceX=off  SenseConstraintForceY=off  SenseConstraintForceZ=off  SenseConstraintTorque=off  SenseConstraintTorqueX=off  SenseConstraintTorqueY=off  SenseConstraintTorqueZ=off  SenseTotalForce=off  SenseTotalForceX=off  SenseTotalForceY=off  SenseTotalForceZ=off  SenseTotalTorque=off  SenseTotalTorqueX=off  SenseTotalTorqueY=off  SenseTotalTorqueZ=off  CompositeWrenchDir=FollowerOnBase  CompositeWrenchFrame=BaseFrame  EquilibriumPosition=0  EquilibriumPositionUnits=rad  SpringStiffness=0  SpringStiffnessUnits=m*N/rad  DampingCoefficient=0  DampingCoefficientUnits=m*s*N/rad  TorqueActuationMode=ComputedTorque  MotionActuationMode=InputMotion  SensePosition=on  SenseVelocity=on  SenseAcceleration=off  SenseTorqueForce=off  PositionTargetSpecify=on  PositionTargetPriority=Low  PositionTargetValue=147.78278879911423  PositionTargetValueUnits=deg  VelocityTargetSpecify=off  VelocityTargetPriority=High  VelocityTargetValue=0  VelocityTargetValueUnits=deg/s
  Simulink-PS Converter1 : nesl_utility/Simulink-PS Converter  PhysicalDomain=network_engine_domain  SubClassName=ps_input  LeftPortType=input  RightPortType=output  PseudoPeriodic=off  Frequencies=[]  NoiseDistribution=none  NoiseParameters=[]  Unit=1  AffineConversion=off  FilteringAndDerivatives=provide  SimscapeFilterOrder=1  InputFilterTimeConstant=0.001  UdotUserProvided=2
  Simulink-PS Converter2 : nesl_utility/Simulink-PS Converter  PhysicalDomain=network_engine_domain  SubClassName=ps_input  LeftPortType=input  RightPortType=output  PseudoPeriodic=off  Frequencies=[]  NoiseDistribution=none  NoiseParameters=[]  Unit=1  AffineConversion=off  FilteringAndDerivatives=provide  SimscapeFilterOrder=1  InputFilterTimeConstant=0.001  UdotUserProvided=2
  Simulink-PS Converter3 : nesl_utility/Simulink-PS Converter  PhysicalDomain=network_engine_domain  SubClassName=ps_input  LeftPortType=input  RightPortType=output  PseudoPeriodic=off  Frequencies=[]  NoiseDistribution=none  NoiseParameters=[]  Unit=1  AffineConversion=off  FilteringAndDerivatives=provide  SimscapeFilterOrder=1  InputFilterTimeConstant=0.001  UdotUserProvided=2
  Solver Configuration : nesl_utility/Solver Configuration  PhysicalDomain=network_engine_domain  SubClassName=solver  LeftPortType=input  RightPortType=generic  Accelerate=off  Tones=[]  Harmonics=[]  SimulateNoise=off  Profile=off  UseLocalSampling=off  EnableSwitchedLinearOptims=on  FrequencyDomain=off  UseCCode=off  RelTol=0.001  AbsTol=1e-06  MinStep=1e-09  ToWorkspace=off  RevertToSquareIcSolve=off  NumHomotopyIterations=100  PhasorMode=off  PhasorModeNumHarmonics=1  OverrideAbsTol=off  DoDC=off  ResidualTolerance=1e-09  UseLocalSolver=off  LocalSolverChoice=NE_BACKWARD_EULER_ADVANCER  LocalSolverSampleTime=0.001  DoFixedCost=off  MaxNonlinIter=3  MaxModeIter=2  LinearAlgebra=Sparse  DelaysMemoryBudget=1024  AutomaticFiltering=on  FilteringTimeConstant=0.001
  Transform : sm_lib/Frames and Transforms/Rigid Transform  TranslationMethod=Cartesian  TranslationStandardOffset=0  TranslationLengthUnit=mm  TranslationStandardAxis=+Z  TranslationCartesianOffset=[3.2381648972062655 30.790535925156188 57.399389346895354]  TranslationROffset=0  TranslationROffsetUnits=m  TranslationZOffset=0  TranslationZOffsetUnits=m  TranslationThetaOffset=0  TranslationThetaOffsetUnits=deg  RotationMethod=ArbitraryAxis  RotationAngleUnits=rad  RotationStandardAxis=+Z  RotationAngle=2.0943951023931913  RotationArbitraryAxis=[0.5773502691896224 0.57735026918963239 0.5773502691896224]  FollAlignAxisA=+X  BaseAlignAxisA=+Y  FollAlignAxisB=+Y  BaseAlignAxisB=+Z  RotationSequenceAxes=FollowerAxes  RotationSequence=XYX  RotationSequenceAngles=[0 0 0]  RotationSequenceAnglesUnits=deg  RotationMatrix=[1 0 0; 0 1 0; 0 0 1]
  World : sm_lib/Frames and Transforms/World Frame
  groud_1_RIGID : Subsystem
  test_pitch_1_RIGID : Subsystem
  test_roll_1_RIGID : Subsystem
  test_yaw_1_RIGID : Subsystem
  "F imu " : PMIOPort  Port=1  Side=Right
  F : PMIOPort  Port=2  Side=Left
  yaw angle out : Outport
  pitch angle out : Outport  Port=2
  roll angle out : Outport  Port=3
  yaw angle v out : Outport  Port=4
  pitch angle v out : Outport  Port=5
  roll angle v out : Outport  Port=6
  wires:
  PS-Simulink Converter1/1 -> yaw angle v out/1
  PS-Simulink Converter3/1 -> pitch angle v out/1
  PS-Simulink Converter/1 -> yaw angle out/1
  PS-Simulink Converter4/1 -> roll angle out/1
  PS-Simulink Converter2/1 -> pitch angle out/1
  PS-Simulink Converter5/1 -> roll angle v out/1
  Derivative2/1 -> Derivative3/1, Simulink-PS Converter2/2
  Derivative3/1 -> Simulink-PS Converter2/3
  Integrator3/1 -> Simulink-PS Converter1/2, Integrator2/1
  Derivative1/1 -> Simulink-PS Converter3/2, Derivative4/1
  Derivative4/1 -> Simulink-PS Converter3/3
  yaw angle acc/1 -> Simulink-PS Converter1/3, Integrator3/1
  roll angle in/1 -> Derivative1/1, Simulink-PS Converter3/1
  pitch angle in/1 -> Derivative2/1, Simulink-PS Converter2/1
  Integrator2/1 -> Simulink-PS Converter1/1
  connections:
  Revolute2/LConn1 -- test_yaw_1_RIGID/RConn1
  Revolute4/LConn1 -- groud_1_RIGID/RConn1
  Revolute3/RConn1 -- test_roll_1_RIGID/LConn2
  Revolute3/LConn1 -- test_pitch_1_RIGID/RConn1
  Revolute4/RConn1 -- test_yaw_1_RIGID/LConn1
  Transform/RConn1 -- groud_1_RIGID/LConn1
  MechanismConfiguration/RConn1 -- Solver Configuration/RConn1 -- World/RConn1 -- "F imu "/RConn1 -- Transform/LConn1
  Revolute2/RConn1 -- test_pitch_1_RIGID/LConn1
  F/RConn1 -- test_roll_1_RIGID/LConn1
  PS-Simulink Converter4/LConn1 -- Revolute3/RConn2
  PS-Simulink Converter1/LConn1 -- Revolute4/RConn3
  PS-Simulink Converter3/LConn1 -- Revolute2/RConn3
  PS-Simulink Converter2/LConn1 -- Revolute2/RConn2
  PS-Simulink Converter5/LConn1 -- Revolute3/RConn3
  Simulink-PS Converter2/RConn1 -- Revolute2/LConn2
  Simulink-PS Converter1/RConn1 -- Revolute4/LConn2
  Simulink-PS Converter3/RConn1 -- Revolute3/LConn2
  PS-Simulink Converter/LConn1 -- Revolute4/RConn2

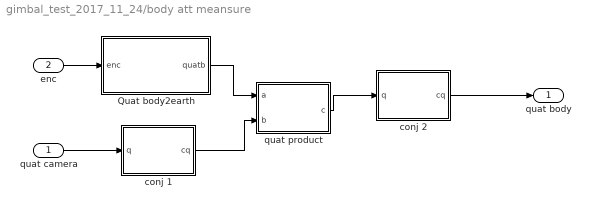
== system gimbal_test_2017_11_24/body att meansure ==
  quat camera : Inport
  enc : Inport  Port=2
  Quat body2earth : MATLAB Function  TreatAsAtomicUnit=on
  conj 1 : MATLAB Function  TreatAsAtomicUnit=on
  conj 2 : MATLAB Function  TreatAsAtomicUnit=on
  "quat product " : MATLAB Function  TreatAsAtomicUnit=on
  quat body : Outport
  wires:
  "quat product "/1(c) -> conj 2/1(q)
  Quat body2earth/1(quatb) -> "quat product "/1(a)
  conj 2/1(cq) -> quat body/1
  enc/1 -> Quat body2earth/1(enc)
  quat camera/1 -> conj 1/1(q)
  conj 1/1(cq) -> "quat product "/2(b)

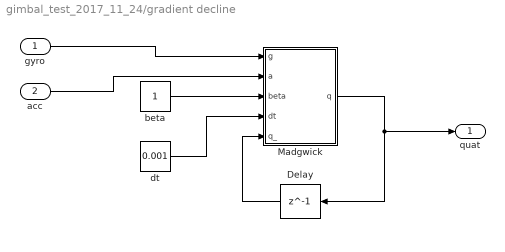
== system gimbal_test_2017_11_24/gradient decline ==
  gyro : Inport
  acc : Inport  Port=2
  Delay : Delay  DelayLength=1  InitialCondition=[1;0;0;0]
  Madgwick : MATLAB Function  TreatAsAtomicUnit=on
  beta : Constant
  dt : Constant  Value=0.001
  quat : Outport
  wires:
  acc/1 -> Madgwick/2(a)
  gyro/1 -> Madgwick/1(g)
  Madgwick/1(q) -> quat/1, Delay/1
  Delay/1 -> Madgwick/5(q_)
  beta/1 -> Madgwick/3(beta)
  dt/1 -> Madgwick/4(dt)

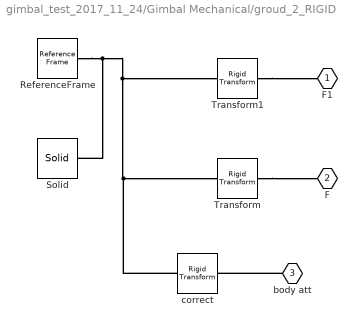
== system gimbal_test_2017_11_24/Gimbal Mechanical/groud_2_RIGID ==
  ReferenceFrame : sm_lib/Frames and Transforms/Reference Frame
  Solid : sm_lib/Body Elements/Solid  InertiaType=Custom  Mass=0.744656095436107  MassUnits=kg  CenterOfMass=[0 14.834199182049298 0]  CenterOfMassUnits=mm  MomentsOfInertia=[248.52962199765179 383.88524366097863 245.75166872905808]  MomentsOfInertiaUnits=kg*mm^2  ProductsOfInertia=[0 0 0]  ProductsOfInertiaUnits=kg*mm^2  DensityBased=on  Density=1000  DensityUnits=kg/(m^3)  DoExposeReferenceFrame=on  SerializedFrames=<Frames/>  GraphicType=FromGeometry  MarkerShape=Sphere  MarkerSize=10  GraphicVisPropType=SimpleVisualProperties  GraphicDiffuseColor=[0.89411764705882346 0.9137254901960784 0.92941176470588238]  GraphicSpecularColor=[0.5 0.5 0.5 1.0]  GraphicAmbientColor=[0.15 0.15 0.15 1.0]  GraphicEmissiveColor=[0.0 0.0 0.0 1.0]  GraphicShininess=75  GraphicOpacity=1  GeometryShape=FromFile  RectangleSize=[1 1]  RectangleSizeUnits=m  BrickDimensions=[1 1 1]  BrickDimensionUnits=m  CylinderRadius=1  CylinderRadiusUnits=m  CylinderLength=1  CylinderLengthUnits=m  SphereRadius=1  SphereRadiusUnits=m  EllipsoidRadii=[1 1 1]  EllipsoidRadiiUnits=m  ExtrusionCrossSection=[1 1; -1 1; -1 -1; 1 -1]  ExtrusionCrossSectionUnits=m  ExtrusionLength=1  ExtrusionLengthUnits=m  PolygonNumSides=3  PolygonOuterRadius=1  PolygonOuterRadiusUnits=m  ExtGeomFileType=STEP  ExtGeomFileName=groud_默认_sldprt.STEP  ExtGeomFileUnits=m  RevolutionCrossSection=[1 1; 1 -1; 2 -1; 2 1]  RevolutionCrossSectionUnits=m  RevolutionExtent=Full  RevolutionAngle=180  RevolutionAngleUnits=deg
  Transform : sm_lib/Frames and Transforms/Rigid Transform  TranslationMethod=Cartesian  TranslationStandardOffset=0  TranslationLengthUnit=mm  TranslationStandardAxis=+Z  TranslationCartesianOffset=[0 30.000000000000028 0]  TranslationROffset=0  TranslationROffsetUnits=m  TranslationZOffset=0  TranslationZOffsetUnits=m  TranslationThetaOffset=0  TranslationThetaOffsetUnits=deg  RotationMethod=ArbitraryAxis  RotationAngleUnits=rad  RotationStandardAxis=+Z  RotationAngle=2.0943951023931953  RotationArbitraryAxis=[0.57735026918962584 -0.57735026918962584 0.57735026918962584]  FollAlignAxisA=+X  BaseAlignAxisA=+Y  FollAlignAxisB=+Y  BaseAlignAxisB=+Z  RotationSequenceAxes=FollowerAxes  RotationSequence=XYX  RotationSequenceAngles=[0 0 0]  RotationSequenceAnglesUnits=deg  RotationMatrix=[1 0 0; 0 1 0; 0 0 1]
  Transform1 : sm_lib/Frames and Transforms/Rigid Transform  TranslationMethod=Cartesian  TranslationStandardOffset=0  TranslationLengthUnit=mm  TranslationStandardAxis=+Z  TranslationCartesianOffset=[-15.000000000000089 49.999999999999453 1.9895196601282805e-13]  TranslationROffset=0  TranslationROffsetUnits=m  TranslationZOffset=0  TranslationZOffsetUnits=m  TranslationThetaOffset=0  TranslationThetaOffsetUnits=deg  RotationMethod=ArbitraryAxis  RotationAngleUnits=rad  RotationStandardAxis=+Z  RotationAngle=3.1415926535897927  RotationArbitraryAxis=[-0 0.70710678118654779 -0.70710678118654746]  FollAlignAxisA=+X  BaseAlignAxisA=+Y  FollAlignAxisB=+Y  BaseAlignAxisB=+Z  RotationSequenceAxes=FollowerAxes  RotationSequence=XYX  RotationSequenceAngles=[0 0 0]  RotationSequenceAnglesUnits=deg  RotationMatrix=[1 0 0; 0 1 0; 0 0 1]
  "correct " : sm_lib/Frames and Transforms/Rigid Transform  TranslationMethod=Cartesian  TranslationStandardOffset=0  TranslationLengthUnit=mm  TranslationStandardAxis=+Z  TranslationCartesianOffset=[0 30.000000000000028 0]  TranslationROffset=0  TranslationROffsetUnits=m  TranslationZOffset=0  TranslationZOffsetUnits=m  TranslationThetaOffset=0  TranslationThetaOffsetUnits=deg  RotationMethod=RotationSequence  RotationAngleUnits=rad  RotationStandardAxis=+Z  RotationAngle=2.0943951023931953  RotationArbitraryAxis=[0.57735026918962584 -0.57735026918962584 0.57735026918962584]  FollAlignAxisA=+X  BaseAlignAxisA=+Y  FollAlignAxisB=+Y  BaseAlignAxisB=+Z  RotationSequenceAxes=BaseAxes  RotationSequence=ZXY  RotationSequenceAngles=[90 -90 0]  RotationSequenceAnglesUnits=deg  RotationMatrix=[1 0 0; 0 1 0; 0 0 1]
  F1 : PMIOPort  Port=1  Side=Left
  F : PMIOPort  Port=2  Side=Right
  "body att " : PMIOPort  Port=3  Side=Right
  connections:
  Solid/RConn1 -- ReferenceFrame/RConn1 -- "correct "/LConn1 -- Transform/LConn1 -- Transform1/LConn1
  Transform/RConn1 -- F/RConn1
  Transform1/RConn1 -- F1/RConn1
  "body att "/RConn1 -- "correct "/RConn1

== system gimbal_test_2017_11_24/Gimbal Mechanical/load_1_RIGID ==
  ReferenceFrame : sm_lib/Frames and Transforms/Reference Frame
  Solid : sm_lib/Body Elements/Solid  InertiaType=Custom  Mass=1  MassUnits=kg  CenterOfMass=[0 59.999999999999993 0]  CenterOfMassUnits=mm  MomentsOfInertia=[1859.7918325794678 2515.5241310829001 3044.0569909542664]  MomentsOfInertiaUnits=kg*mm^2  ProductsOfInertia=[0 0 0]  ProductsOfInertiaUnits=kg*mm^2  DensityBased=on  Density=1000  DensityUnits=kg/(m^3)  DoExposeReferenceFrame=on  SerializedFrames=<Frames/>  GraphicType=FromGeometry  MarkerShape=Sphere  MarkerSize=10  GraphicVisPropType=SimpleVisualProperties  GraphicDiffuseColor=[0.89803921568627454 0.91764705882352937 0.92941176470588238]  GraphicSpecularColor=[0.5 0.5 0.5 1.0]  GraphicAmbientColor=[0.15 0.15 0.15 1.0]  GraphicEmissiveColor=[0.0 0.0 0.0 1.0]  GraphicShininess=75  GraphicOpacity=1  GeometryShape=FromFile  RectangleSize=[1 1]  RectangleSizeUnits=m  BrickDimensions=[1 1 1]  BrickDimensionUnits=m  CylinderRadius=1  CylinderRadiusUnits=m  CylinderLength=1  CylinderLengthUnits=m  SphereRadius=1  SphereRadiusUnits=m  EllipsoidRadii=[1 1 1]  EllipsoidRadiiUnits=m  ExtrusionCrossSection=[1 1; -1 1; -1 -1; 1 -1]  ExtrusionCrossSectionUnits=m  ExtrusionLength=1  ExtrusionLengthUnits=m  PolygonNumSides=3  PolygonOuterRadius=1  PolygonOuterRadiusUnits=m  ExtGeomFileType=STEP  ExtGeomFileName=load_默认_sldprt.STEP  ExtGeomFileUnits=m  RevolutionCrossSection=[1 1; 1 -1; 2 -1; 2 1]  RevolutionCrossSectionUnits=m  RevolutionExtent=Full  RevolutionAngle=180  RevolutionAngleUnits=deg
  Transform : sm_lib/Frames and Transforms/Rigid Transform  TranslationMethod=Cartesian  TranslationStandardOffset=0  TranslationLengthUnit=mm  TranslationStandardAxis=+Z  TranslationCartesianOffset=[-153.63399999999999 -5.6843418860808015e-13 31.999999999999623]  TranslationROffset=0  TranslationROffsetUnits=m  TranslationZOffset=0  TranslationZOffsetUnits=m  TranslationThetaOffset=0  TranslationThetaOffsetUnits=deg  RotationMethod=ArbitraryAxis  RotationAngleUnits=rad  RotationStandardAxis=+Z  RotationAngle=2.0943951023931944  RotationArbitraryAxis=[-0.57735026918962584 0.57735026918962629 0.57735026918962518]  FollAlignAxisA=+X  BaseAlignAxisA=+Y  FollAlignAxisB=+Y  BaseAlignAxisB=+Z  RotationSequenceAxes=FollowerAxes  RotationSequence=XYX  RotationSequenceAngles=[0 0 0]  RotationSequenceAnglesUnits=deg  RotationMatrix=[1 0 0; 0 1 0; 0 0 1]
  F : PMIOPort  Port=1  Side=Left
  connections:
  Solid/RConn1 -- ReferenceFrame/RConn1 -- Transform/LConn1
  Transform/RConn1 -- F/RConn1
